simulink model "non-linear"  (R2014b)
settings: Solver=ode3  StartTime=0.0  StopTime=30  FixedStep=0.1  RelTol=1e-3
values from neighbouring files (symbols this model uses):
  b = 0.002    [params.m]
  d = 11.8/100    (= 0.118)    [params.m]
  g = 9.812    [params.m]
  L = place(A',C',[po1 po2])'    [params.m]    (also in state-space.m = place(A',C',[ob1 ob2])')
  m = 2/1000    (= 0.002)    [params.m]
settings Model: Creator=mtsou_000  LastModifiedBy=mtsou_000

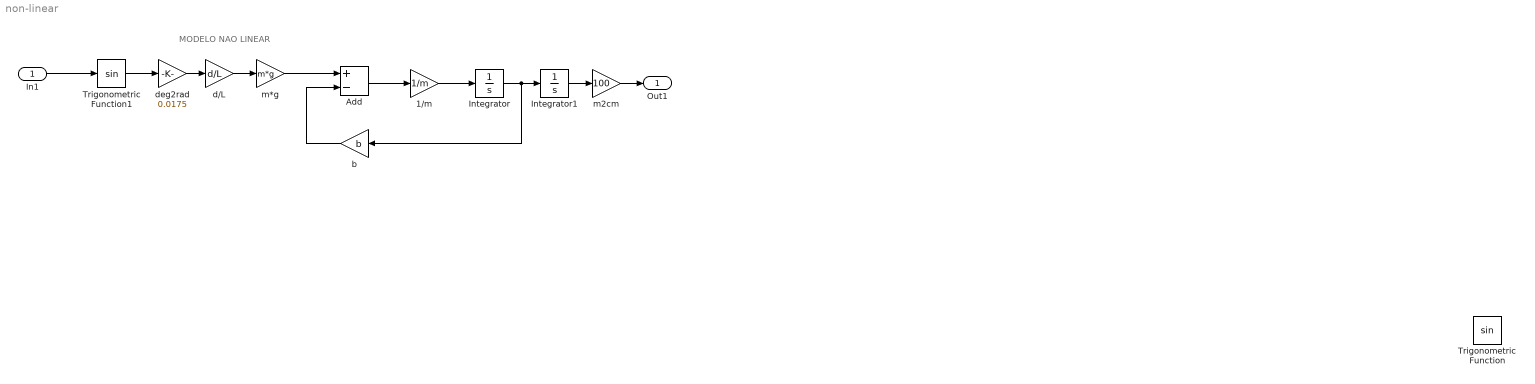
== system non-linear ==
  note: MODELO NAO LINEAR
  In1 : Inport
  1/m : Gain  Gain=1/m
  Add : Sum  Inputs=+-
  Integrator : Integrator
  Integrator1 : Integrator  InitialCondition=.05
  Trigonometric Function : Trigonometry
  Trigonometric Function1 : Trigonometry
  b : Gain  Gain=b
  d/L : Gain  Gain=d/L
  deg2rad : Gain  Gain=0.0175
  m*g : Gain  Gain=m*g
  m2cm : Gain  Gain=100
  Out1 : Outport
  wires:
  b/1 -> Add/2
  Add/1 -> 1/m/1
  m*g/1 -> Add/1
  1/m/1 -> Integrator/1
  Integrator/1 -> b/1, Integrator1/1
  Integrator1/1 -> m2cm/1
  m2cm/1 -> Out1/1
  deg2rad/1 -> d/L/1
  d/L/1 -> m*g/1
  In1/1 -> Trigonometric Function1/1
  Trigonometric Function1/1 -> deg2rad/1
